simulink subsystem "ros_command"  (R2021a)
settings: Solver=VariableStepAuto  StartTime=0.0  StopTime=10.0  RelTol=1e-3
undefined symbols (not defined in the file): MPC
libraries: robotlib x5
settings Model: Creator=lamarre  LastModifiedBy=lamarre

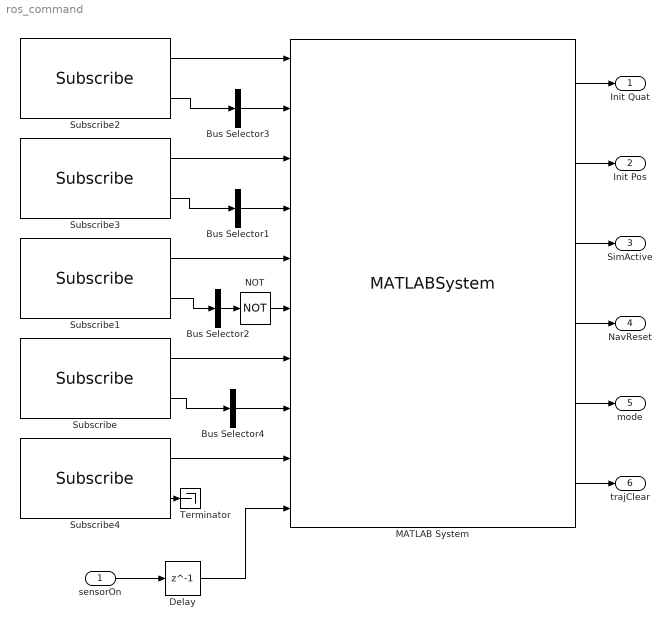
== system ros_command ==
  sensorOn : Inport
  Bus Selector1 : BusSelector  OutputSignals=Data  OutputAsBus=on
  Bus Selector2 : BusSelector  OutputSignals=State  OutputAsBus=on
  Bus Selector3 : BusSelector  OutputSignals=Data  OutputAsBus=on
  Bus Selector4 : BusSelector  OutputSignals=Position.X,Position.Y,Position.Z,Orientation.W,Orientation.X,Orientation.Y,Orientation.Z  OutputAsBus=on
  Delay : Delay  DelayLength=1  InitialCondition=0
  MATLAB System : MATLABSystem  System=rosCommandManager  initial_mode=0  SimulateUsing=Code generation
      mask Type: rosCommandManager
      mask Display:
      | disp('rosCommandManager');
      | port_label('input',1,'newSetMode');
      | port_label('input',2,'setMode');
      | port_label('input',3,'newReset');
      | port_label('input',4,'reset');
      | port_label('input',5,'newKill');
      | port_label('input',6,'kill');
      | port_label('input',7,'newIc');
      | port_label('input',8,'ic');
      | port_label('input',9,'newTrajreset');
      | port_label('input',10,'sensorOn');
      | port_label('output',1,'initQuat');
      | port_label('output',2,'initPos');
      | port_label('output',3,'simEnable');
      | port_label('output',4,'reset');
      | port_label('output',5,'mode');
      | port_label('output',6,'trajClear');
  NOT : Logic  Operator=NOT  IconShape=distinctive  AllPortsSameDT=off  OutDataTypeStr=boolean
  Subscribe : robotlib/Subscribe  topicSource=Select from ROS network  topic=/initial_condition  messageType=geometry_msgs/Pose  SampleTime=MPC.Ts  legacyBusStruct=off  messageQueueLength=1
  Subscribe1 : robotlib/Subscribe  topicSource=Specify your own  topic=/provider_kill_mission/kill_switch_msg  messageType=sonia_common/KillSwitchMsg  SampleTime=MPC.Ts  legacyBusStruct=off  messageQueueLength=1
  Subscribe2 : robotlib/Subscribe  topicSource=Specify your own  topic=/proc_control/set_mode  messageType=std_msgs/UInt8  SampleTime=MPC.Ts  legacyBusStruct=off  messageQueueLength=1
  Subscribe3 : robotlib/Subscribe  topicSource=Specify your own  topic=/proc_nav/reset_pos  messageType=std_msgs/Bool  SampleTime=MPC.Ts  legacyBusStruct=off  messageQueueLength=1
  Subscribe4 : robotlib/Subscribe  topicSource=Specify your own  topic=/proc_control/reset_trajectory  messageType=std_msgs/Bool  SampleTime=MPC.Ts  legacyBusStruct=off  messageQueueLength=1
  Terminator : Terminator
  Init Quat : Outport
  Init Pos : Outport  Port=2
  SimActive : Outport  Port=3
  NavReset : Outport  Port=4
  mode : Outport  Port=5
  trajClear : Outport  Port=6
  wires:
  Subscribe2/2 -> Bus Selector3/1
  Bus Selector3/1 -> MATLAB System/2
  Subscribe3/1 -> MATLAB System/3
  Subscribe3/2 -> Bus Selector1/1
  Subscribe1/1 -> MATLAB System/5
  Subscribe1/2 -> Bus Selector2/1
  Subscribe/1 -> MATLAB System/7
  Subscribe/2 -> Bus Selector4/1
  MATLAB System/5 -> mode/1
  Subscribe2/1 -> MATLAB System/1
  Bus Selector1/1 -> MATLAB System/4
  Bus Selector4/1 -> MATLAB System/8
  MATLAB System/4 -> NavReset/1
  MATLAB System/3 -> SimActive/1
  MATLAB System/6 -> trajClear/1
  MATLAB System/1 -> Init Quat/1
  MATLAB System/2 -> Init Pos/1
  Bus Selector2/1 -> NOT/1
  NOT/1 -> MATLAB System/6
  sensorOn/1 -> Delay/1
  Delay/1 -> MATLAB System/10
  Subscribe4/1 -> MATLAB System/9
  Subscribe4/2 -> Terminator/1
